simulink model "simulink_2f"  (R2020b)
settings: Solver=VariableStepAuto  StartTime=0.0  StopTime=500  RelTol=1e-3
values from neighbouring files (symbols this model uses):
  A_c = [-0.322   0.052   0.028  -1.12    0.002 ... (first row only)    [task_2_f.m]
  B_c = [0 ... (first row only)    [task_2_f.m]
  C_c = [1 0 0 0 0 ... (first row only)    [task_2_f.m]
  d_chi = 1.5*deg2rad    (= 0.0261799387799)    [task_2.m]    (also in task_2_f.m)
  g = 9.81    [task_2.m]    (also in task_2_f.m)
  k_d_phi = (2*zeta_phi*w_phi_n - a_phi_1)/a_phi_2    [task_2.m]    (also in task_2_f.m)
  k_i_chi = w_n_chi^2*V_g/g    [task_2.m]    (also in task_2_f.m)
  k_p_chi = 2*zeta_chi*w_n_chi*V_g/g    [task_2.m]    (also in task_2_f.m)
  k_p_phi = delta_a_max/e_phi_max * sign(a_phi_2)    [task_2.m]    (also in task_2_f.m)
  V_g = 540/3.6    (= 150)    [task_2.m]    (also in task_2_f.m)
libraries: simulink x1
settings Model: Creator=dino  LastModifiedBy=Øystein Solbø
settings DataIOCC: ReturnWorkspaceOutputs=off
settings DebuggingCC: ArithmeticOperatorsInVariantConditions=warning
settings SFSimCC: CustomCodeUndefinedFunction=UseInterfaceOnly

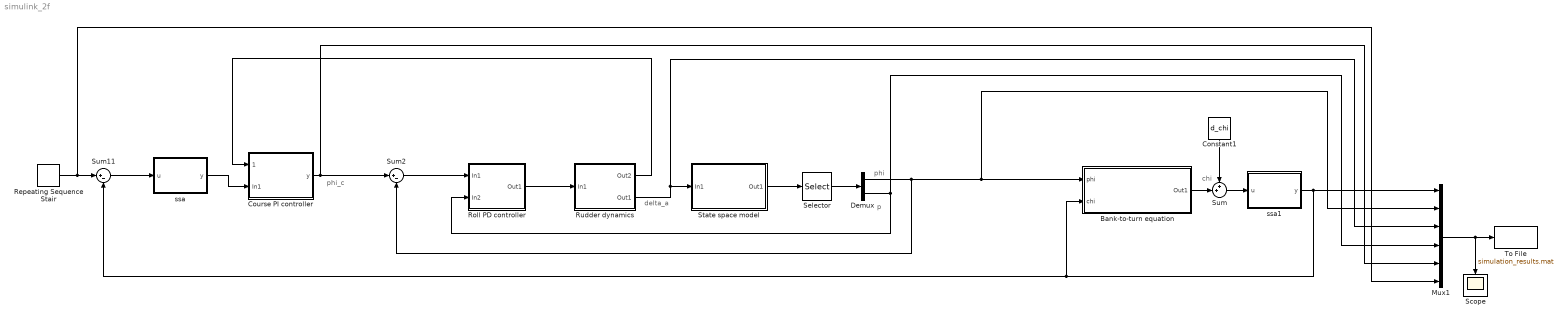
== system simulink_2f ==
  note: delta_a
  note: p
  note: phi
  note: chi
  note: phi_c
  Bank-to-turn equation : Subsystem
  Constant1 : Constant  Value=d_chi
  Course PI controller : Subsystem
  Demux : Demux  Outputs=2
  Mux1 : Mux  Inputs=6
  Repeating Sequence Stair : simulink/Sources/Repeating Sequence Stair  OutValues=chi_ref_step.'  tsamp=-1  OutMin=[]  OutMax=[]  OutDataTypeStr=double  OutputDataTypeScalingMode=double  OutDataType=fixdt(0,8)  ConRadixGroup=Best Precision: Vector-wise  OutScaling=2^-12
  Roll PD controller : Subsystem
  Rudder dynamics : Subsystem
  Scope : Scope
  Selector : Selector  InputPortWidth=4  IndexOptions=Index vector (dialog)  Indices=[2 3]  OutputSizes=1
  State space model : Subsystem
  Sum : Sum  Inputs=++|
  Sum11 : Sum  Inputs=|+-
  Sum2 : Sum  Inputs=|+-
  To File : ToFile  Filename=simulation_results.mat
  ssa : MATLAB Function  TreatAsAtomicUnit=on
  ssa1 : MATLAB Function  TreatAsAtomicUnit=on
  wires:
  Sum11/1 -> ssa/1(u)
  Repeating Sequence Stair/1 -> Sum11/1, Mux1/6
  Mux1/1 -> To File/1, Scope/1
  Sum/1 -> ssa1/1(u)
  Course PI controller/1(y) -> Sum2/1, Mux1/5
  ssa/1(y) -> Course PI controller/2(In1)
  State space model/1(Out1) -> Selector/1
  Selector/1 -> Demux/1
  Rudder dynamics/2(Out1) -> Mux1/3, State space model/1(In1)
  Constant1/1 -> Sum/1
  Demux/2 -> Roll PD controller/2(In2), Mux1/4
  Bank-to-turn equation/1(Out1) -> Sum/2
  Demux/1 -> Mux1/2, Bank-to-turn equation/1(phi), Sum2/2
  Sum2/1 -> Roll PD controller/1(In1)
  Roll PD controller/1(Out1) -> Rudder dynamics/1(In1)
  ssa1/1(y) -> Sum11/2, Bank-to-turn equation/2(chi), Mux1/1
  Rudder dynamics/1(Out2) -> Course PI controller/1(" ")

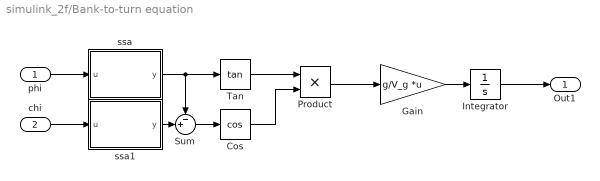
== system simulink_2f/Bank-to-turn equation ==
  phi : Inport
  chi : Inport  Port=2
  Cos : Trigonometry  Operator=cos
  Gain : Gain  Gain=g/V_g  Multiplication=Matrix(K*u)
  Integrator : Integrator
  Product : Product
  Sum : Sum  Inputs=-+|
  Tan : Trigonometry  Operator=tan
  ssa : MATLAB Function  TreatAsAtomicUnit=on
  ssa1 : MATLAB Function  TreatAsAtomicUnit=on
  Out1 : Outport
  wires:
  Integrator/1 -> Out1/1
  Gain/1 -> Integrator/1
  Product/1 -> Gain/1
  phi/1 -> ssa/1(u)
  Cos/1 -> Product/2
  Tan/1 -> Product/1
  Sum/1 -> Cos/1
  ssa/1(y) -> Sum/1, Tan/1
  ssa1/1(y) -> Sum/2
  chi/1 -> ssa1/1(u)

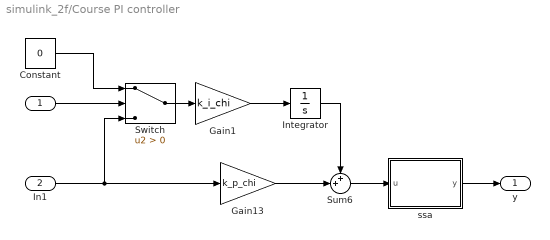
== system simulink_2f/Course PI controller ==
  " " : Inport
  In1 : Inport  Port=2
  Constant : Constant  Value=0
  Gain1 : Gain  Gain=k_i_chi
  Gain13 : Gain  Gain=k_p_chi
  Integrator : Integrator
  Sum6 : Sum  Inputs=++|
  Switch : Switch  Criteria=u2 > Threshold
  ssa : MATLAB Function  TreatAsAtomicUnit=on
  y : Outport
  wires:
  In1/1 -> Switch/3, Gain13/1
  Integrator/1 -> Sum6/1
  Gain1/1 -> Integrator/1
  Gain13/1 -> Sum6/2
  Sum6/1 -> ssa/1(u)
  ssa/1(y) -> y/1
  Switch/1 -> Gain1/1
  " "/1 -> Switch/2
  Constant/1 -> Switch/1

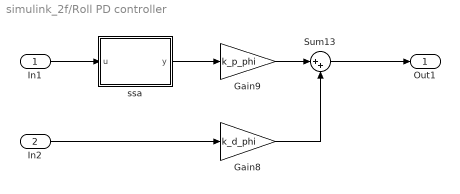
== system simulink_2f/Roll PD controller ==
  In1 : Inport
  In2 : Inport  Port=2
  Gain8 : Gain  Gain=k_d_phi
  Gain9 : Gain  Gain=k_p_phi
  Sum13 : Sum  Inputs=|++
  ssa : MATLAB Function  TreatAsAtomicUnit=on
  Out1 : Outport
  wires:
  Gain9/1 -> Sum13/1
  In1/1 -> ssa/1(u)
  Sum13/1 -> Out1/1
  In2/1 -> Gain8/1
  Gain8/1 -> Sum13/2
  ssa/1(y) -> Gain9/1

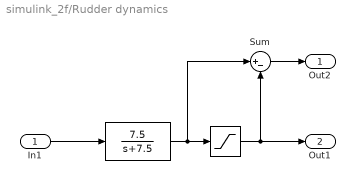
== system simulink_2f/Rudder dynamics ==
  In1 : Inport
  " " : TransferFcn  Numerator=[0 7.5]  Denominator=[1 7.5]
  " " : Saturate  UpperLimit=30*deg2rad  LowerLimit=-30*deg2rad
  Sum : Sum  Inputs=|+-
  Out2 : Outport
  Out1 : Outport  Port=2
  wires:
  In1/1 -> " "/1
  " "/1 -> Sum/1, " "/1
  " "/1 -> Sum/2, Out1/1
  Sum/1 -> Out2/1

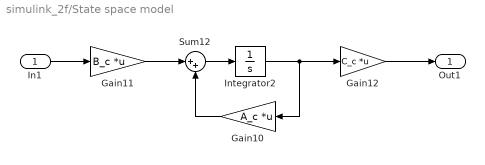
== system simulink_2f/State space model ==
  In1 : Inport
  Gain10 : Gain  Gain=A_c  Multiplication=Matrix(K*u)
  Gain11 : Gain  Gain=B_c  Multiplication=Matrix(K*u)
  Gain12 : Gain  Gain=C_c  Multiplication=Matrix(K*u)
  Integrator2 : Integrator
  Sum12 : Sum  Inputs=|++
  Out1 : Outport
  wires:
  Gain10/1 -> Sum12/2
  Sum12/1 -> Integrator2/1
  Gain11/1 -> Sum12/1
  In1/1 -> Gain11/1
  Integrator2/1 -> Gain10/1, Gain12/1
  Gain12/1 -> Out1/1

== matlab function simulink_2f/Course PI controller/ssa ==
  data: u input; y output
function y = fcn(u)
y = ssa(u);

== matlab function simulink_2f/Roll PD controller/ssa ==
  data: u input; y output
function y = fcn(u)
y = ssa(u);

== matlab function simulink_2f/Bank-to-turn equation/ssa ==
  data: u input; y output
function y = fcn(u)
y = ssa(u);

== matlab function simulink_2f/Bank-to-turn equation/ssa1 ==
  data: u input; y output
function y = fcn(u)
y = ssa(u);

== matlab function simulink_2f/ssa1 ==
  data: u input; y output
function y = fcn(u)
y = ssa(u);

== matlab function simulink_2f/ssa ==
  data: u input; y output
function y = fcn(u)
y = ssa(u);
